simulink model "flightControlSystem"  (R2024a)
settings: Solver=ode3  StartTime=0  StopTime=TFinal  FixedStep=Ts  RelTol=1e-3  EnableMultiTasking=on
undefined symbols (not defined in the file): codertarget, Controller, DiscIntNeverNeededParam, Discrete, Estimator, g, init, orient_ref, pos_ref, Sensors, Time, Ts, var_acc_angle_N, var_bias_gyr_N, var_gyro_p_N, Vehicle
libraries: simulink x125, slpidlib x35, ctrlSharedLib x12, sharedtransform x10, eeGeneralControl x8, parrotlib x6, shareduavrstlib x1, simulink_need_slupdate x1
(part 9 of 11)

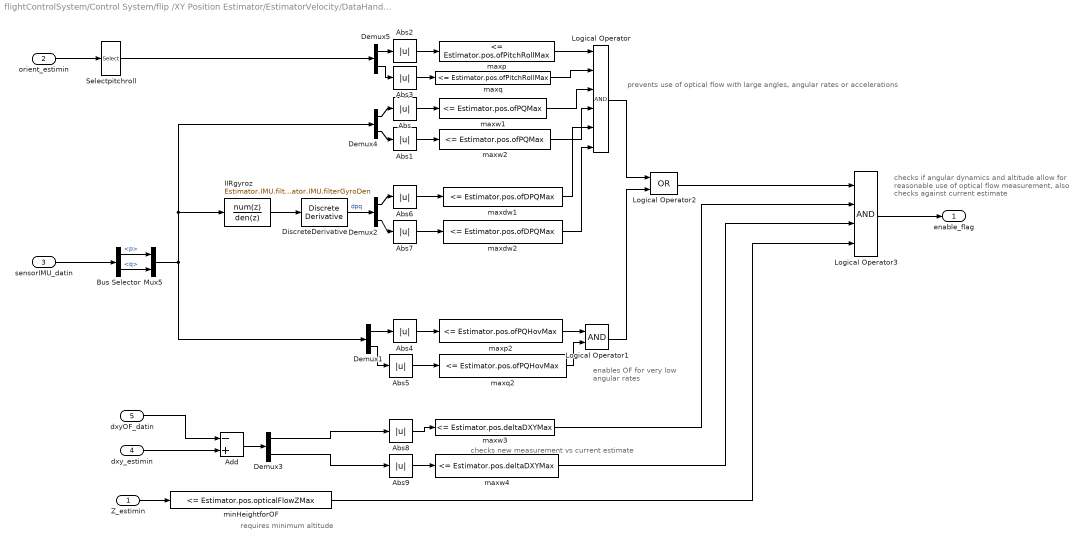
== system flightControlSystem/Control System/flip /XY Position Estimator/EstimatorVelocity/DataHandling ==
  note: prevents use of optical flow with large angles, angular rates or accelerations
  note: enables OF for very
      | low angular rates
  note: checks if angular dynamics and altitude allow for
      | reasonable use of optical flow measurement,
      | also checks against current estimate
  note: checks new measurement vs current estimate
  note: requires minimum altitude
  Z_estimin : Inport
  orient_estimin : Inport  Port=2
  sensorIMU_datin : Inport  Port=3
  dxy_estimin : Inport  Port=4
  dxyOF_datin : Inport  Port=5
  Abs{,1..9} (10 alike) : Abs  SaturateOnIntegerOverflow=off
  Add : Sum  Inputs=-+
  Bus Selector : BusSelector  OutputSignals=p,q
  Demux{1..5} (5 alike) : Demux  Outputs=2
  DiscreteDerivative : simulink/Discrete/Discrete Derivative  gainval=1.0  ICPrevScaledInput=0.0  OutMin=[]  OutMax=[]  OutDataType=fixdt(1, 16)  OutScaling=2^-10  DoSatur=off
  IIRgyroz : DiscreteFilter  Numerator=Estimator.IMU.filterGyroNum  Denominator=Estimator.IMU.filterGyroDen
  Logical Operator : Logic  Inputs=6  AllPortsSameDT=off  OutDataTypeStr=boolean
  Logical Operator1 : Logic  AllPortsSameDT=off  OutDataTypeStr=boolean
  Logical Operator2 : Logic  Operator=OR  AllPortsSameDT=off  OutDataTypeStr=boolean
  Logical Operator3 : Logic  Inputs=4  AllPortsSameDT=off  OutDataTypeStr=boolean
  Mux5 : Mux  Inputs=2
  Selectpitchroll : Selector  InputPortWidth=3  IndexOptions=Index vector (dialog)  Indices=[2 3]  OutputSizes=1
  maxdw1 : simulink/Logic and Bit Operations/Compare To Constant  relop=<=  const=Estimator.pos.ofDPQMax  OutDataTypeStr=boolean
  maxdw2 : simulink/Logic and Bit Operations/Compare To Constant  relop=<=  const=Estimator.pos.ofDPQMax  OutDataTypeStr=boolean
  maxp : simulink/Logic and Bit Operations/Compare To Constant  relop=<=  const=Estimator.pos.ofPitchRollMax  OutDataTypeStr=boolean
  maxp2 : simulink/Logic and Bit Operations/Compare To Constant  relop=<=  const=Estimator.pos.ofPQHovMax  OutDataTypeStr=boolean
  maxq : simulink/Logic and Bit Operations/Compare To Constant  relop=<=  const=Estimator.pos.ofPitchRollMax  OutDataTypeStr=boolean
  maxq2 : simulink/Logic and Bit Operations/Compare To Constant  relop=<=  const=Estimator.pos.ofPQHovMax  OutDataTypeStr=boolean
  maxw1 : simulink/Logic and Bit Operations/Compare To Constant  relop=<=  const=Estimator.pos.ofPQMax  OutDataTypeStr=boolean
  maxw2 : simulink/Logic and Bit Operations/Compare To Constant  relop=<=  const=Estimator.pos.ofPQMax  OutDataTypeStr=boolean
  maxw3 : simulink/Logic and Bit Operations/Compare To Constant  relop=<=  const=Estimator.pos.deltaDXYMax  OutDataTypeStr=boolean
  maxw4 : simulink/Logic and Bit Operations/Compare To Constant  relop=<=  const=Estimator.pos.deltaDXYMax  OutDataTypeStr=boolean
  minHeightforOF : simulink/Logic and Bit Operations/Compare To Constant  relop=<=  const=Estimator.pos.opticalFlowZMax  OutDataTypeStr=boolean
  enable_flag : Outport  VectorParamsAs1DForOutWhenUnconnected=off
  wires:
  minHeightforOF/1 -> Logical Operator3/4
  IIRgyroz/1 -> DiscreteDerivative/1
  Mux5/1 -> Demux1/1, Demux4/1, IIRgyroz/1
  maxw4/1 -> Logical Operator3/3
  maxw3/1 -> Logical Operator3/2
  dxyOF_datin/1 -> Add/1
  Demux3/2 -> Abs9/1
  Demux3/1 -> Abs8/1
  dxy_estimin/1 -> Add/2
  Add/1 -> Demux3/1
  Abs9/1 -> maxw4/1
  Abs8/1 -> maxw3/1
  Logical Operator2/1 -> Logical Operator3/1
  Logical Operator3/1 -> enable_flag/1
  DiscreteDerivative/1 -> Demux2/1  "dpq"
  Demux2/2 -> Abs7/1
  Demux2/1 -> Abs6/1
  Abs7/1 -> maxdw2/1
  Abs6/1 -> maxdw1/1
  Logical Operator1/1 -> Logical Operator2/2
  Demux1/2 -> Abs5/1
  Demux1/1 -> Abs4/1
  Abs5/1 -> maxq2/1
  Abs4/1 -> maxp2/1
  Abs3/1 -> maxq/1
  Abs2/1 -> maxp/1
  Demux4/2 -> Abs1/1
  Demux4/1 -> Abs/1
  Abs1/1 -> maxw2/1
  Abs/1 -> maxw1/1
  Z_estimin/1 -> minHeightforOF/1
  Logical Operator/1 -> Logical Operator2/1
  maxw1/1 -> Logical Operator/3
  Bus Selector/1 -> Mux5/1  "<p>"
  Selectpitchroll/1 -> Demux5/1
  sensorIMU_datin/1 -> Bus Selector/1
  maxq2/1 -> Logical Operator1/2
  Bus Selector/2 -> Mux5/2  "<q>"
  maxp/1 -> Logical Operator/1
  maxw2/1 -> Logical Operator/4
  orient_estimin/1 -> Selectpitchroll/1
  maxdw1/1 -> Logical Operator/5
  maxdw2/1 -> Logical Operator/6
  maxq/1 -> Logical Operator/2
  Demux5/1 -> Abs2/1
  Demux5/2 -> Abs3/1
  maxp2/1 -> Logical Operator1/1

== system flightControlSystem/Control System/flip /XY Position Estimator/EstimatorVelocity/XY velocity w//o angular velocity compensation ==
  note: Optical flow raw readings are converted to velocity in m/s based on the estimated altitude
  optical_flow : Inport
  z_estimate : Inport  Port=2
  " " : Product  Inputs=**
  Compare To Constant : simulink/Logic and Bit Operations/Compare To Constant  relop=<  const=200*4  OutDataTypeStr=boolean
  Counter Free-Running : simulink/Sources/Counter Free-Running  NumBits=32  tsamp=-1
  Gain : Gain  Gain=-1
  Select dxy : Selector  InputPortWidth=3  IndexOptions=Index vector (dialog)  Indices=[1 2]  OutputSizes=1
  Switch : Switch  Criteria=u2 > Threshold  SaturateOnIntegerOverflow=off  InputSameDT=off
  opticalFlowErrorCorrect : Gain  Gain=1.15
  optical_flow_dx_dy : Outport
  wires:
  Select dxy/1 -> optical_flow_dx_dy/1  "optical_flow_dx_dy"
  " "/1 -> opticalFlowErrorCorrect/1
  opticalFlowErrorCorrect/1 -> Switch/3
  Gain/1 -> " "/2
  Switch/1 -> Select dxy/1
  Counter Free-Running/1 -> Compare To Constant/1
  Compare To Constant/1 -> Switch/2
  optical_flow/1 -> " "/1, Switch/1
  z_estimate/1 -> Gain/1

== system flightControlSystem/Control System/normal/SensorPreprocessing/Temperature Compensation/Triggered Subsystem ==
  In1 : Inport
  Trigger : TriggerPort  TriggerType=either  VariantControl=Variant
  Out1 : Outport
  wires:
  In1/1 -> Out1/1

== system flightControlSystem/Control System/normal/XY Position Estimator/EstimatorVelocity/AccelerationHandling ==
  dxy_estimin : Inport
  sensorIMU_datin : Inport  Port=2
  orient_estimin : Inport  Port=3
  Z_estimin : Inport  Port=4
  Add : Sum  Inputs=-+
  Bus Selector1 : BusSelector  OutputSignals=ddx,ddy,ddz
  Deactivate Acceleration If OF is not used due to low altitude : simulink/Logic and Bit Operations/Compare To Constant  relop=<=  const=Estimator.pos.opticalFlowZMax  OutDataTypeStr=boolean
  Logical Operator : Logic  Operator=OR  AllPortsSameDT=off  OutDataTypeStr=boolean
  Mux6 : Mux  Inputs=3
  Product : Product  Inputs=3
  Product1 : Product  Multiplication=Matrix(*)
  Rotation Angles to Direction Cosine Matrix : sharedtransform/Rotation Angles to Direction Cosine Matrix  rotationOrder=ZYX  aMode=aMode
  SelectPlanarddxy : Selector  InputPortWidth=3  IndexOptions=Index vector (dialog)  Indices=[1 2]  OutputSizes=1
  Selector : Selector  InputPortWidth=2  IndexOptions=Index vector (dialog)  Indices=1  OutputSizes=1
  Selector1 : Selector  InputPortWidth=2  IndexOptions=Index vector (dialog)  Indices=2  OutputSizes=1
  do not use acc if optical flow never available (Note OF@60Hz but ZOH to 200!) : simulink/Logic and Bit Operations/Compare To Constant  relop=~=  const=0  OutDataTypeStr=boolean
  do not use acc if optical flow never available (Note OF@60Hz but ZOH to 200!)1 : simulink/Logic and Bit Operations/Compare To Constant  relop=~=  const=0  OutDataTypeStr=boolean
  gainaccinput1 : Gain  OutDataTypeStr=single
  gravity : Constant  Value=[0 0 -g]
  acceleration_world : Outport  OutDataTypeStr=single  VectorParamsAs1DForOutWhenUnconnected=off
  wires:
  do not use acc if optical flow never available (Note OF@60Hz but ZOH to 200!)1/1 -> Logical Operator/2
  do not use acc if optical flow never available (Note OF@60Hz but ZOH to 200!)/1 -> Logical Operator/1
  Logical Operator/1 -> Product/1
  Selector1/1 -> do not use acc if optical flow never available (Note OF@60Hz but ZOH to 200!)1/1
  Selector/1 -> do not use acc if optical flow never available (Note OF@60Hz but ZOH to 200!)/1
  dxy_estimin/1 -> Selector1/1, Selector/1
  Product/1 -> acceleration_world/1
  Deactivate Acceleration If OF is not used due to low altitude/1 -> Product/3
  Z_estimin/1 -> Deactivate Acceleration If OF is not used due to low altitude/1
  Add/1 -> SelectPlanarddxy/1
  Product1/1 -> Add/1
  gravity/1 -> Product1/2
  SelectPlanarddxy/1 -> gainaccinput1/1
  Bus Selector1/3 -> Mux6/3  "<ddz>"
  Bus Selector1/1 -> Mux6/1  "<ddx>"
  sensorIMU_datin/1 -> Bus Selector1/1
  Mux6/1 -> Add/2
  Bus Selector1/2 -> Mux6/2  "<ddy>"
  orient_estimin/1 -> Rotation Angles to Direction Cosine Matrix/1
  Rotation Angles to Direction Cosine Matrix/1 -> Product1/1
  gainaccinput1/1 -> Product/2

== system flightControlSystem/Control System/normal/XY Position Estimator/EstimatorVelocity/Angular velocity compensation for optical flow ==
  note: Optical flow readings are affected by both linear and angular velocity of the drone. We need to subtract the effect of angular velocity before using the flow data
  z_estimate : Inport
  Angular velocity w/o bias : Inport  Port=2
  Abs : Abs  SaturateOnIntegerOverflow=off
  Data Type Conversion : DataTypeConversion  SaturateOnIntegerOverflow=off  RndMeth=Floor
  Demux : Demux  Outputs=2
  Gain1 : Gain  Gain=-1
  Mux : Mux  Inputs=2
  Selector : Selector  InputPortWidth=3  IndexOptions=Index vector (dialog)  Indices=[1 2]  OutputSizes=1
  prod : Product  Inputs=**
  angular velocity correction : Outport
  wires:
  Gain1/1 -> Mux/1
  Mux/1 -> Data Type Conversion/1
  Demux/2 -> Gain1/1
  Data Type Conversion/1 -> angular velocity correction/1
  prod/1 -> Demux/1
  z_estimate/1 -> Abs/1
  Demux/1 -> Mux/2
  Selector/1 -> prod/2
  Abs/1 -> prod/1
  Angular velocity w/o bias/1 -> Selector/1

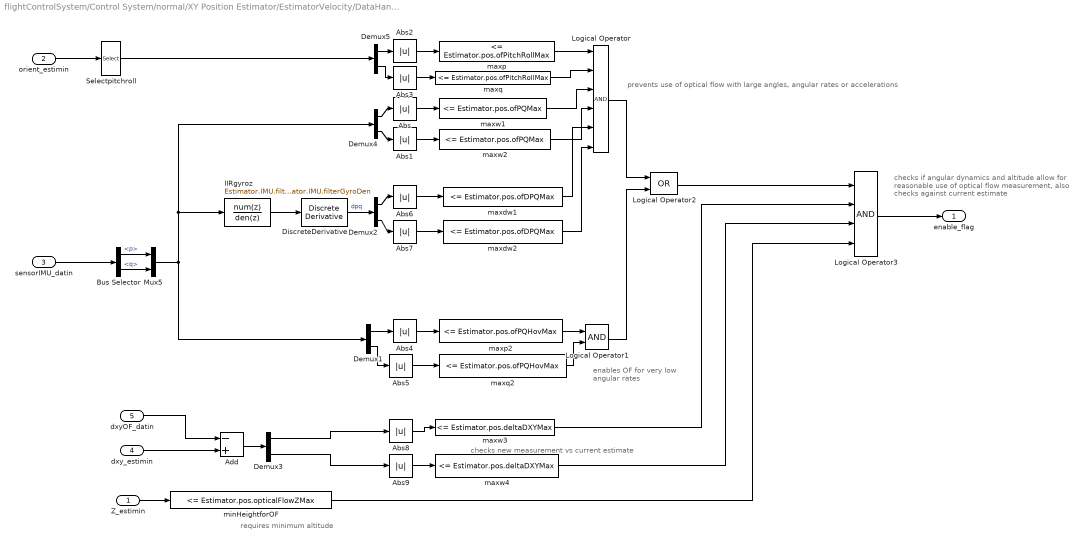
== system flightControlSystem/Control System/normal/XY Position Estimator/EstimatorVelocity/DataHandling ==
  note: prevents use of optical flow with large angles, angular rates or accelerations
  note: enables OF for very
      | low angular rates
  note: checks if angular dynamics and altitude allow for
      | reasonable use of optical flow measurement,
      | also checks against current estimate
  note: checks new measurement vs current estimate
  note: requires minimum altitude
  Z_estimin : Inport
  orient_estimin : Inport  Port=2
  sensorIMU_datin : Inport  Port=3
  dxy_estimin : Inport  Port=4
  dxyOF_datin : Inport  Port=5
  Abs{,1..9} (10 alike) : Abs  SaturateOnIntegerOverflow=off
  Add : Sum  Inputs=-+
  Bus Selector : BusSelector  OutputSignals=p,q
  Demux{1..5} (5 alike) : Demux  Outputs=2
  DiscreteDerivative : simulink/Discrete/Discrete Derivative  gainval=1.0  ICPrevScaledInput=0.0  OutMin=[]  OutMax=[]  OutDataType=fixdt(1, 16)  OutScaling=2^-10  DoSatur=off
  IIRgyroz : DiscreteFilter  Numerator=Estimator.IMU.filterGyroNum  Denominator=Estimator.IMU.filterGyroDen
  Logical Operator : Logic  Inputs=6  AllPortsSameDT=off  OutDataTypeStr=boolean
  Logical Operator1 : Logic  AllPortsSameDT=off  OutDataTypeStr=boolean
  Logical Operator2 : Logic  Operator=OR  AllPortsSameDT=off  OutDataTypeStr=boolean
  Logical Operator3 : Logic  Inputs=4  AllPortsSameDT=off  OutDataTypeStr=boolean
  Mux5 : Mux  Inputs=2
  Selectpitchroll : Selector  InputPortWidth=3  IndexOptions=Index vector (dialog)  Indices=[2 3]  OutputSizes=1
  maxdw1 : simulink/Logic and Bit Operations/Compare To Constant  relop=<=  const=Estimator.pos.ofDPQMax  OutDataTypeStr=boolean
  maxdw2 : simulink/Logic and Bit Operations/Compare To Constant  relop=<=  const=Estimator.pos.ofDPQMax  OutDataTypeStr=boolean
  maxp : simulink/Logic and Bit Operations/Compare To Constant  relop=<=  const=Estimator.pos.ofPitchRollMax  OutDataTypeStr=boolean
  maxp2 : simulink/Logic and Bit Operations/Compare To Constant  relop=<=  const=Estimator.pos.ofPQHovMax  OutDataTypeStr=boolean
  maxq : simulink/Logic and Bit Operations/Compare To Constant  relop=<=  const=Estimator.pos.ofPitchRollMax  OutDataTypeStr=boolean
  maxq2 : simulink/Logic and Bit Operations/Compare To Constant  relop=<=  const=Estimator.pos.ofPQHovMax  OutDataTypeStr=boolean
  maxw1 : simulink/Logic and Bit Operations/Compare To Constant  relop=<=  const=Estimator.pos.ofPQMax  OutDataTypeStr=boolean
  maxw2 : simulink/Logic and Bit Operations/Compare To Constant  relop=<=  const=Estimator.pos.ofPQMax  OutDataTypeStr=boolean
  maxw3 : simulink/Logic and Bit Operations/Compare To Constant  relop=<=  const=Estimator.pos.deltaDXYMax  OutDataTypeStr=boolean
  maxw4 : simulink/Logic and Bit Operations/Compare To Constant  relop=<=  const=Estimator.pos.deltaDXYMax  OutDataTypeStr=boolean
  minHeightforOF : simulink/Logic and Bit Operations/Compare To Constant  relop=<=  const=Estimator.pos.opticalFlowZMax  OutDataTypeStr=boolean
  enable_flag : Outport  VectorParamsAs1DForOutWhenUnconnected=off
  wires:
  minHeightforOF/1 -> Logical Operator3/4
  IIRgyroz/1 -> DiscreteDerivative/1
  Mux5/1 -> Demux1/1, Demux4/1, IIRgyroz/1
  maxw4/1 -> Logical Operator3/3
  maxw3/1 -> Logical Operator3/2
  dxyOF_datin/1 -> Add/1
  Demux3/2 -> Abs9/1
  Demux3/1 -> Abs8/1
  dxy_estimin/1 -> Add/2
  Add/1 -> Demux3/1
  Abs9/1 -> maxw4/1
  Abs8/1 -> maxw3/1
  Logical Operator2/1 -> Logical Operator3/1
  Logical Operator3/1 -> enable_flag/1
  DiscreteDerivative/1 -> Demux2/1  "dpq"
  Demux2/2 -> Abs7/1
  Demux2/1 -> Abs6/1
  Abs7/1 -> maxdw2/1
  Abs6/1 -> maxdw1/1
  Logical Operator1/1 -> Logical Operator2/2
  Demux1/2 -> Abs5/1
  Demux1/1 -> Abs4/1
  Abs5/1 -> maxq2/1
  Abs4/1 -> maxp2/1
  Abs3/1 -> maxq/1
  Abs2/1 -> maxp/1
  Demux4/2 -> Abs1/1
  Demux4/1 -> Abs/1
  Abs1/1 -> maxw2/1
  Abs/1 -> maxw1/1
  Z_estimin/1 -> minHeightforOF/1
  Logical Operator/1 -> Logical Operator2/1
  maxw1/1 -> Logical Operator/3
  Bus Selector/1 -> Mux5/1  "<p>"
  Selectpitchroll/1 -> Demux5/1
  sensorIMU_datin/1 -> Bus Selector/1
  maxq2/1 -> Logical Operator1/2
  Bus Selector/2 -> Mux5/2  "<q>"
  maxp/1 -> Logical Operator/1
  maxw2/1 -> Logical Operator/4
  orient_estimin/1 -> Selectpitchroll/1
  maxdw1/1 -> Logical Operator/5
  maxdw2/1 -> Logical Operator/6
  maxq/1 -> Logical Operator/2
  Demux5/1 -> Abs2/1
  Demux5/2 -> Abs3/1
  maxp2/1 -> Logical Operator1/1

== system flightControlSystem/Control System/normal/XY Position Estimator/EstimatorVelocity/xy velocity w//o angular velocity compensation ==
  note: Optical flow raw readings are converted to velocity in m/s based on the estimated altitude
  optical_flow : Inport
  z_estimate : Inport  Port=2
  " " : Product  Inputs=**
  Compare To Constant : simulink/Logic and Bit Operations/Compare To Constant  relop=<  const=200*4  OutDataTypeStr=boolean
  Counter Free-Running : simulink/Sources/Counter Free-Running  NumBits=32  tsamp=-1
  Gain : Gain  Gain=-1
  Select dxy : Selector  InputPortWidth=3  IndexOptions=Index vector (dialog)  Indices=[1 2]  OutputSizes=1
  Switch : Switch  Criteria=u2 > Threshold  SaturateOnIntegerOverflow=off  InputSameDT=off
  opticalFlowErrorCorrect : Gain  Gain=1.15
  optical_flow_dx_dy : Outport
  wires:
  Select dxy/1 -> optical_flow_dx_dy/1  "optical_flow_dx_dy"
  " "/1 -> opticalFlowErrorCorrect/1
  opticalFlowErrorCorrect/1 -> Switch/3
  Gain/1 -> " "/2
  Switch/1 -> Select dxy/1
  Counter Free-Running/1 -> Compare To Constant/1
  Compare To Constant/1 -> Switch/2
  optical_flow/1 -> " "/1, Switch/1
  z_estimate/1 -> Gain/1

== system flightControlSystem/Flight Control System/State Estimator/SensorPreprocessing/Temperature Compensation/Triggered Subsystem ==
  In1 : Inport
  Trigger : TriggerPort  TriggerType=either  VariantControl=Variant
  Out1 : Outport
  wires:
  In1/1 -> Out1/1

== system flightControlSystem/Flight Control System/State Estimator/XY Position Estimator/EstimatorVelocity/AccelerationHandling ==
  dxy_estimin : Inport
  sensorIMU_datin : Inport  Port=2
  orient_estimin : Inport  Port=3
  Z_estimin : Inport  Port=4
  Add : Sum  Inputs=-+
  Bus Selector1 : BusSelector  OutputSignals=ddx,ddy,ddz
  Deactivate Acceleration If OF is not used due to low altitude : simulink/Logic and Bit Operations/Compare To Constant  relop=<=  const=Estimator.pos.opticalFlowZMax  OutDataTypeStr=boolean
  Logical Operator : Logic  Operator=OR  AllPortsSameDT=off  OutDataTypeStr=boolean
  Mux6 : Mux  Inputs=3
  Product : Product  Inputs=3
  Product1 : Product  Multiplication=Matrix(*)
  Rotation Angles to Direction Cosine Matrix : sharedtransform/Rotation Angles to Direction Cosine Matrix  rotationOrder=ZYX  aMode=aMode
  SelectPlanarddxy : Selector  InputPortWidth=3  IndexOptions=Index vector (dialog)  Indices=[1 2]  OutputSizes=1
  Selector : Selector  InputPortWidth=2  IndexOptions=Index vector (dialog)  Indices=1  OutputSizes=1
  Selector1 : Selector  InputPortWidth=2  IndexOptions=Index vector (dialog)  Indices=2  OutputSizes=1
  do not use acc if optical flow never available (Note OF@60Hz but ZOH to 200!) : simulink/Logic and Bit Operations/Compare To Constant  relop=~=  const=0  OutDataTypeStr=boolean
  do not use acc if optical flow never available (Note OF@60Hz but ZOH to 200!)1 : simulink/Logic and Bit Operations/Compare To Constant  relop=~=  const=0  OutDataTypeStr=boolean
  gainaccinput1 : Gain  OutDataTypeStr=single
  gravity : Constant  Value=[0 0 -g]
  acceleration_world : Outport  OutDataTypeStr=single  VectorParamsAs1DForOutWhenUnconnected=off
  wires:
  do not use acc if optical flow never available (Note OF@60Hz but ZOH to 200!)1/1 -> Logical Operator/2
  do not use acc if optical flow never available (Note OF@60Hz but ZOH to 200!)/1 -> Logical Operator/1
  Logical Operator/1 -> Product/1
  Selector1/1 -> do not use acc if optical flow never available (Note OF@60Hz but ZOH to 200!)1/1
  Selector/1 -> do not use acc if optical flow never available (Note OF@60Hz but ZOH to 200!)/1
  dxy_estimin/1 -> Selector1/1, Selector/1
  Product/1 -> acceleration_world/1
  Deactivate Acceleration If OF is not used due to low altitude/1 -> Product/3
  Z_estimin/1 -> Deactivate Acceleration If OF is not used due to low altitude/1
  Add/1 -> SelectPlanarddxy/1
  Product1/1 -> Add/1
  gravity/1 -> Product1/2
  SelectPlanarddxy/1 -> gainaccinput1/1
  Bus Selector1/3 -> Mux6/3  "<ddz>"
  Bus Selector1/1 -> Mux6/1  "<ddx>"
  sensorIMU_datin/1 -> Bus Selector1/1
  Mux6/1 -> Add/2
  Bus Selector1/2 -> Mux6/2  "<ddy>"
  orient_estimin/1 -> Rotation Angles to Direction Cosine Matrix/1
  Rotation Angles to Direction Cosine Matrix/1 -> Product1/1
  gainaccinput1/1 -> Product/2

== system flightControlSystem/Flight Control System/State Estimator/XY Position Estimator/EstimatorVelocity/Angular velocity compensation for optical flow ==
  note: Optical flow readings are affected by both linear and angular velocity of the drone. We need to subtract the effect of angular velocity before using the flow data
  z_estimate : Inport
  Angular velocity w/o bias : Inport  Port=2
  Abs : Abs  SaturateOnIntegerOverflow=off
  Data Type Conversion : DataTypeConversion  SaturateOnIntegerOverflow=off  RndMeth=Floor
  Demux : Demux  Outputs=2
  Gain1 : Gain  Gain=-1
  Mux : Mux  Inputs=2
  Selector : Selector  InputPortWidth=3  IndexOptions=Index vector (dialog)  Indices=[1 2]  OutputSizes=1
  prod : Product  Inputs=**
  angular velocity correction : Outport
  wires:
  Gain1/1 -> Mux/1
  Mux/1 -> Data Type Conversion/1
  Demux/2 -> Gain1/1
  Data Type Conversion/1 -> angular velocity correction/1
  prod/1 -> Demux/1
  z_estimate/1 -> Abs/1
  Demux/1 -> Mux/2
  Selector/1 -> prod/2
  Abs/1 -> prod/1
  Angular velocity w/o bias/1 -> Selector/1

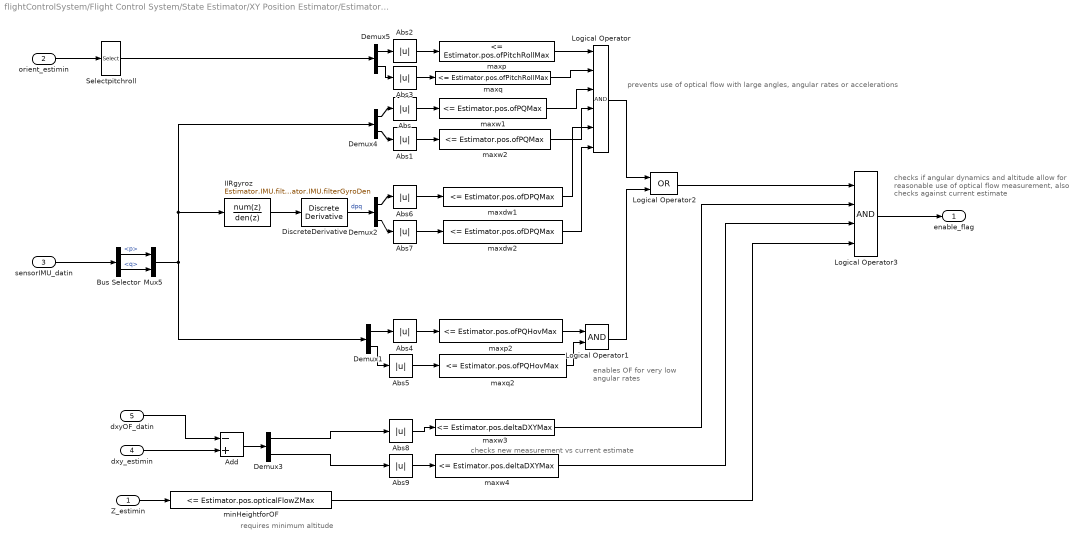
== system flightControlSystem/Flight Control System/State Estimator/XY Position Estimator/EstimatorVelocity/DataHandling ==
  note: prevents use of optical flow with large angles, angular rates or accelerations
  note: enables OF for very
      | low angular rates
  note: checks if angular dynamics and altitude allow for
      | reasonable use of optical flow measurement,
      | also checks against current estimate
  note: checks new measurement vs current estimate
  note: requires minimum altitude
  Z_estimin : Inport
  orient_estimin : Inport  Port=2
  sensorIMU_datin : Inport  Port=3
  dxy_estimin : Inport  Port=4
  dxyOF_datin : Inport  Port=5
  Abs{,1..9} (10 alike) : Abs  SaturateOnIntegerOverflow=off
  Add : Sum  Inputs=-+
  Bus Selector : BusSelector  OutputSignals=p,q
  Demux{1..5} (5 alike) : Demux  Outputs=2
  DiscreteDerivative : simulink/Discrete/Discrete Derivative  gainval=1.0  ICPrevScaledInput=0.0  OutMin=[]  OutMax=[]  OutDataType=fixdt(1, 16)  OutScaling=2^-10  DoSatur=off
  IIRgyroz : DiscreteFilter  Numerator=Estimator.IMU.filterGyroNum  Denominator=Estimator.IMU.filterGyroDen
  Logical Operator : Logic  Inputs=6  AllPortsSameDT=off  OutDataTypeStr=boolean
  Logical Operator1 : Logic  AllPortsSameDT=off  OutDataTypeStr=boolean
  Logical Operator2 : Logic  Operator=OR  AllPortsSameDT=off  OutDataTypeStr=boolean
  Logical Operator3 : Logic  Inputs=4  AllPortsSameDT=off  OutDataTypeStr=boolean
  Mux5 : Mux  Inputs=2
  Selectpitchroll : Selector  InputPortWidth=3  IndexOptions=Index vector (dialog)  Indices=[2 3]  OutputSizes=1
  maxdw1 : simulink/Logic and Bit Operations/Compare To Constant  relop=<=  const=Estimator.pos.ofDPQMax  OutDataTypeStr=boolean
  maxdw2 : simulink/Logic and Bit Operations/Compare To Constant  relop=<=  const=Estimator.pos.ofDPQMax  OutDataTypeStr=boolean
  maxp : simulink/Logic and Bit Operations/Compare To Constant  relop=<=  const=Estimator.pos.ofPitchRollMax  OutDataTypeStr=boolean
  maxp2 : simulink/Logic and Bit Operations/Compare To Constant  relop=<=  const=Estimator.pos.ofPQHovMax  OutDataTypeStr=boolean
  maxq : simulink/Logic and Bit Operations/Compare To Constant  relop=<=  const=Estimator.pos.ofPitchRollMax  OutDataTypeStr=boolean
  maxq2 : simulink/Logic and Bit Operations/Compare To Constant  relop=<=  const=Estimator.pos.ofPQHovMax  OutDataTypeStr=boolean
  maxw1 : simulink/Logic and Bit Operations/Compare To Constant  relop=<=  const=Estimator.pos.ofPQMax  OutDataTypeStr=boolean
  maxw2 : simulink/Logic and Bit Operations/Compare To Constant  relop=<=  const=Estimator.pos.ofPQMax  OutDataTypeStr=boolean
  maxw3 : simulink/Logic and Bit Operations/Compare To Constant  relop=<=  const=Estimator.pos.deltaDXYMax  OutDataTypeStr=boolean
  maxw4 : simulink/Logic and Bit Operations/Compare To Constant  relop=<=  const=Estimator.pos.deltaDXYMax  OutDataTypeStr=boolean
  minHeightforOF : simulink/Logic and Bit Operations/Compare To Constant  relop=<=  const=Estimator.pos.opticalFlowZMax  OutDataTypeStr=boolean
  enable_flag : Outport  VectorParamsAs1DForOutWhenUnconnected=off
  wires:
  minHeightforOF/1 -> Logical Operator3/4
  IIRgyroz/1 -> DiscreteDerivative/1
  Mux5/1 -> Demux1/1, Demux4/1, IIRgyroz/1
  maxw4/1 -> Logical Operator3/3
  maxw3/1 -> Logical Operator3/2
  dxyOF_datin/1 -> Add/1
  Demux3/2 -> Abs9/1
  Demux3/1 -> Abs8/1
  dxy_estimin/1 -> Add/2
  Add/1 -> Demux3/1
  Abs9/1 -> maxw4/1
  Abs8/1 -> maxw3/1
  Logical Operator2/1 -> Logical Operator3/1
  Logical Operator3/1 -> enable_flag/1
  DiscreteDerivative/1 -> Demux2/1  "dpq"
  Demux2/2 -> Abs7/1
  Demux2/1 -> Abs6/1
  Abs7/1 -> maxdw2/1
  Abs6/1 -> maxdw1/1
  Logical Operator1/1 -> Logical Operator2/2
  Demux1/2 -> Abs5/1
  Demux1/1 -> Abs4/1
  Abs5/1 -> maxq2/1
  Abs4/1 -> maxp2/1
  Abs3/1 -> maxq/1
  Abs2/1 -> maxp/1
  Demux4/2 -> Abs1/1
  Demux4/1 -> Abs/1
  Abs1/1 -> maxw2/1
  Abs/1 -> maxw1/1
  Z_estimin/1 -> minHeightforOF/1
  Logical Operator/1 -> Logical Operator2/1
  maxw1/1 -> Logical Operator/3
  Bus Selector/1 -> Mux5/1  "<p>"
  Selectpitchroll/1 -> Demux5/1
  sensorIMU_datin/1 -> Bus Selector/1
  maxq2/1 -> Logical Operator1/2
  Bus Selector/2 -> Mux5/2  "<q>"
  maxp/1 -> Logical Operator/1
  maxw2/1 -> Logical Operator/4
  orient_estimin/1 -> Selectpitchroll/1
  maxdw1/1 -> Logical Operator/5
  maxdw2/1 -> Logical Operator/6
  maxq/1 -> Logical Operator/2
  Demux5/1 -> Abs2/1
  Demux5/2 -> Abs3/1
  maxp2/1 -> Logical Operator1/1

== system flightControlSystem/Flight Control System/State Estimator/XY Position Estimator/EstimatorVelocity/xy velocity w//o angular velocity compensation ==
  note: Optical flow raw readings are converted to velocity in m/s based on the estimated altitude
  optical_flow : Inport
  z_estimate : Inport  Port=2
  " " : Product  Inputs=**
  Compare To Constant : simulink/Logic and Bit Operations/Compare To Constant  relop=<  const=200*4  OutDataTypeStr=boolean
  Counter Free-Running : simulink/Sources/Counter Free-Running  NumBits=32  tsamp=-1
  Gain : Gain  Gain=-1
  Select dxy : Selector  InputPortWidth=3  IndexOptions=Index vector (dialog)  Indices=[1 2]  OutputSizes=1
  Switch : Switch  Criteria=u2 > Threshold  SaturateOnIntegerOverflow=off  InputSameDT=off
  opticalFlowErrorCorrect : Gain  Gain=1.15
  optical_flow_dx_dy : Outport
  wires:
  Select dxy/1 -> optical_flow_dx_dy/1  "optical_flow_dx_dy"
  " "/1 -> opticalFlowErrorCorrect/1
  opticalFlowErrorCorrect/1 -> Switch/3
  Gain/1 -> " "/2
  Switch/1 -> Select dxy/1
  Counter Free-Running/1 -> Compare To Constant/1
  Compare To Constant/1 -> Switch/2
  optical_flow/1 -> " "/1, Switch/1
  z_estimate/1 -> Gain/1

== matlab function flightControlSystem/Control System/flip /Attitude Estimator/MATLAB Function1 ==
  data: acc input; q output; gyro input; prevQuat input
function q = fcn(acc, gyro, prevQuat)
    
    
    kcorr = 0.002;
    
    w = norm(gyro);
    
    sigmaW = 0.5 * [0 -gyro';...
        gyro(1) 0 gyro(3) -gyro(2);...
        gyro(2) -gyro(3) 0 gyro(1);...
        gyro(3) gyro(2) -gyro(1) 0];
    
    if w==0
        qpred = prevQuat;
    else
        qpred = (eye(4)*cos(w*0.0025) + (2/w)* sigmaW * sin(w*0.0025))*prevQuat;
    end
    
    if (w < 1) && (abs(norm(acc)-9.81) < 2.9)
        
        qpred = quaternion(qpred');

        accW = rotateframe(conj(qpred),acc');
        
        accW = accW/norm(accW);
        
        epred = [0,0,-1];

        beta = acos(epred*accW');

        hB = cross(accW',epred');

        hB = hB / norm(hB);

        qcorr = quaternion([cos(kcorr*beta/2), hB'*sin(kcorr*beta/2)]);

        qpred = qcorr * qpred;

        [a,b,c,d] = qpred.parts;
        
        qpred = [a,b,c,d]';
    end
    
q =  qpred;
end

== matlab function flightControlSystem/Control System/flip/MATLAB Function ==
  data: t input; w_d output; ap_ input
function w_d = fcn(t, ap_)

w_d = 0;
wmax = 1600*pi/180;
% g1 = pi/wmax;
% b1 = -3/4 * wmax;
% 
% if t > 10 && t < 10.25
%     w_d = (t-10) * wmax/0.25;
% elseif t >= 10.25 && t < 10.5
%     w_d = -(t-10)*wmax/0.25 + 2*wmax;
% end


if t > 10 && t < 10.2287
    w_d = wmax;
elseif t >= 10.2287 && t < 10.2856
    w_d = -(t-10)*wmax/0.0569 + 5.0193*wmax;
end

if ap_ > 360
    w_d = 0;
end

== matlab function flightControlSystem/Control System/flip/Position Controller/Position error transformation (Earth to Body frame) ==
  data: yaw input; xy_err_earth input; xy_err_body output
function xy_err_body = fcn(yaw,xy_err_earth)

transformation = [cos(yaw), sin(yaw); -sin(yaw),  cos(yaw)];
xy_err_body = transformation * xy_err_earth;


end

== matlab function flightControlSystem/Control System/Path Planning/Subsystem3/MATLAB Function2 ==
  data: data input; x_new input; xdd_des output; y_new input; xd_new input; yd_new input; ydd_des output; xdd_new input; ydd_new input; x input; y input; dx input; dy input; ddx input; ddy input
function [xdd_des, ydd_des] = fcn(data, x_new, y_new, xd_new, yd_new, xdd_new, ydd_new, x, y, dx, dy, ddx, ddy)
    % PID gains
    kpx = single(0.0001);
    kpy = single(0.0001);
    kdx = single(0.00001);
    kdy = single(0.00001);

    % Compute desired accelerations
    xdd_des = single(0.0000031 * (xdd_new - ddx) + kdx * (xd_new - dx) + kpx * (x_new - x));
    ydd_des = single(0.0000031 * (ydd_new - ddy) + kdy * (yd_new - dy) + kpy * (y_new - y));
end

== matlab function flightControlSystem/Control System/Path Planning/Subsystem3/MATLAB Function3 ==
  data: xdd_des input; phi_des output; ydd_des input; psi input; theta_des output
function [phi_des, theta_des] = fcn(xdd_des, ydd_des, psi)
    g = 9.81;
    phi_des = single(1/g * (xdd_des * sin(psi) - ydd_des * cos(psi)));
    theta_des = single(-1/g * (xdd_des * cos(psi) + ydd_des * sin(psi)));
end

== stateflow chart flightControlSystem/Control System/Path Planning/Subsystem3/Chart1 ==
  state Hover
    entry:
    phi=0.0;
    theta=0.0;
  state phi_des
    phi=phi_des
    theta=theta_des
  (default) -> Hover
  Hover -> phi_des : [after(2,sec)]
  data: theta_des input; phi_des input; phi output double; theta output double

== stateflow chart flightControlSystem/Control System/Path Planning/Chart1 ==
  state MoveStraight
    during:
    xout=xout+0.006*x_new
    yout=yout+0.006*y_new
    zout=zout;
  state Hover
    entry:
    xout=0.0;
    yout=0.0;
    zout=-0.8;
  state MoveStraight4
    during:
    xout=xout+0.006*x_new;
    yout=yout+0.006*y_new;
    zout=zout+0.0000014*(sum_pixels)
  state land
    finaland=1
  (default) -> Hover
  Hover -> MoveStraight : [after(2,sec)]
  MoveStraight -> MoveStraight4 : [sum_pixels>60&&centroid_dist<25]
  MoveStraight4 -> land : [ zout>-0.4]
  data: ang input; sum_pixels input; centroid_dist input; forward input; right input; left input; sum_pix2 input; xestim input; yestim input; y_new input; xout output single; yout output single; zout output single; x_new input; dy input; dx input; s local; finaland output

== matlab function flightControlSystem/Control System/Path Planning/MATLAB Function2 ==
  data: u input; forward output; right output
function [forward,right]= fcn(u)

forward = u(1);
right=u(2);

== matlab function flightControlSystem/Control System/Controller/Position Controller/MATLAB Function1 ==
  data: ddx input; ddy input; ddx_filtered output; ddz input; ddy_filtered output; ddz_filtered output
function [ddx_filtered, ddy_filtered, ddz_filtered] = fcn(ddx, ddy, ddz)
    persistent filterInitialized b a;
    noise_margin = 0.005; % Define the margin around zero to be considered as noise
    
    if isempty(filterInitialized)
        % Design the filter according to your specifications
        % Example: 2nd-order Butterworth low-pass filter with a cutoff frequency of 5 Hz and a sample rate of 100 Hz
        
        [b, a] = butter(2, (7/(100/2)), 'low');
        filterInitialized = true;
    end
    
    % Apply the filter to each acceleration component
    ddx_temp = filter(b, a, ddx);
    ddy_temp = filter(b, a, ddy);
    ddz_temp = filter(b, a, ddz);

    % Apply the bias correction (deadzone)
    ddx_filtered = applyDeadzone(ddx_temp, noise_margin);
    ddy_filtered = applyDeadzone(ddy_temp, noise_margin);
    ddz_filtered = applyDeadzone(ddz_temp, noise_margin);
end

function val_filtered = applyDeadzone(val, margin)
    % Ensure that the function outputs the same type as the input
    if abs(val) < margin
        val_filtered = cast(0, 'like', val); % Cast zero to the type of val
    else
        val_filtered = val;
    end
end

== matlab function flightControlSystem/Control System/Controller/Position Controller/Position error transformation (Earth to Body frame)1 ==
  data: yaw input; xy_err_earth input; xy_err_body output
function xy_err_body = fcn(yaw,xy_err_earth)

transformation = [cos(yaw), sin(yaw); -sin(yaw),  cos(yaw)];
xy_err_body = transformation * xy_err_earth;


end

== matlab function flightControlSystem/Control System/Controller/Position Controller/Subsystem/MATLAB Function2 ==
  data: Xe input; xdd_des output; Ve input; Ae input; qd input; ydd_des output; q input; qdd input; Je input; qddd input
function [xdd_des, ydd_des] = fcn(Xe,Ve,Ae,qd,q,qdd, Je, qddd)


%Xe actual position x y z
%Ve ACtual velocity Ve(1) Ve(2) Ve(3)
%k2;dx=  kpz=

kpx=1.77;
kpy=1.77;
kpz=75;

kdx=3.4
kdy=3.4
kdz=45

kax=0.01;
kay=0.01;
kaz=0.01;

kjx=0.0002;
kjy=0.0002;
kjz=0.0002;

xdd_des=kjx*(qddd(1))+kax*(qdd(1)-Ae(1))+kdx*(qd(1)-Ve(1))+kpx*(q(1)-Xe(1))
ydd_des=kjy*(qddd(2))+kay*(qdd(2)-Ae(2))+kdy*(qd(2)-Ve(2))+kpy*(q(2)-Xe(2))
%zdd_des=kjz*(qddd(3))+kaz*(qdd(3)-Ae(3))+kdz*(qd(3)-Ve(3))+kpz*(q(3)-Xe(3))



end

== matlab function flightControlSystem/Control System/Controller/Position Controller/Subsystem/MATLAB Function3 ==
  data: u input; y output; u1 input; time input; t output
function [y ,t]= fcn(u, u1, time)



y=[u(1) u1(1);u(2) u1(2) ; u(3) u1(3)]

t=[time time+0.05]
 
end

== matlab function flightControlSystem/Control System/Controller/Position Controller/MATLAB Function2 ==
  data: ddx input; ddy input; ddx_filtered output; ddz input; ddy_filtered output; ddz_filtered output
function [ddx_filtered, ddy_filtered, ddz_filtered] = fcn(ddx, ddy, ddz)
    persistent filterInitialized b a;
    noise_margin = 0.005; % Define the margin around zero to be considered as noise
    
    if isempty(filterInitialized)
        % Design the filter according to your specifications
        % Example: 2nd-order Butterworth low-pass filter with a cutoff frequency of 5 Hz and a sample rate of 100 Hz
        
        [b, a] = butter(2, (7/(100/2)), 'low');
        filterInitialized = true;
    end
    
    % Apply the filter to each acceleration component
    ddx_temp = filter(b, a, ddx);
    ddy_temp = filter(b, a, ddy);
    ddz_temp = filter(b, a, ddz);

    % Apply the bias correction (deadzone)
    ddx_filtered = applyDeadzone(ddx_temp, noise_margin);
    ddy_filtered = applyDeadzone(ddy_temp, noise_margin);
    ddz_filtered = applyDeadzone(ddz_temp, noise_margin);
end

function val_filtered = applyDeadzone(val, margin)
    % Ensure that the function outputs the same type as the input
    if abs(val) < margin
        val_filtered = cast(0, 'like', val); % Cast zero to the type of val
    else
        val_filtered = val;
    end
end

== matlab function flightControlSystem/Control System/Controller/Position Controller/Position error transformation (Earth to Body frame)2 ==
  data: yaw input; xy_err_earth input; xy_err_body output
function xy_err_body = fcn(yaw,xy_err_earth)

transformation = [cos(yaw), sin(yaw); -sin(yaw),  cos(yaw)];
xy_err_body = transformation * xy_err_earth;


end

== matlab function flightControlSystem/Control System/Controller/Position Controller/MATLAB Function3 ==
  data: ddx input; ddy input; ddx_filtered output; ddz input; ddy_filtered output; ddz_filtered output
function [ddx_filtered, ddy_filtered, ddz_filtered] = fcn(ddx, ddy, ddz)
    persistent filterInitialized b a;
    noise_margin = 0.005; % Define the margin around zero to be considered as noise
    
    if isempty(filterInitialized)
        % Design the filter according to your specifications
        % Example: 2nd-order Butterworth low-pass filter with a cutoff frequency of 5 Hz and a sample rate of 100 Hz
        
        [b, a] = butter(2, (7/(100/2)), 'low');
        filterInitialized = true;
    end
    
    % Apply the filter to each acceleration component
    ddx_temp = filter(b, a, ddx);
    ddy_temp = filter(b, a, ddy);
    ddz_temp = filter(b, a, ddz);

    % Apply the bias correction (deadzone)
    ddx_filtered = applyDeadzone(ddx_temp, noise_margin);
    ddy_filtered = applyDeadzone(ddy_temp, noise_margin);
    ddz_filtered = applyDeadzone(ddz_temp, noise_margin);
end

function val_filtered = applyDeadzone(val, margin)
    % Ensure that the function outputs the same type as the input
    if abs(val) < margin
        val_filtered = cast(0, 'like', val); % Cast zero to the type of val
    else
        val_filtered = val;
    end
end

== matlab function flightControlSystem/Control System/Controller/Position Controller/Position error transformation (Earth to Body frame)3 ==
  data: yaw input; xy_err_earth input; xy_err_body output
function xy_err_body = fcn(yaw,xy_err_earth)

transformation = [cos(yaw), sin(yaw); -sin(yaw),  cos(yaw)];
xy_err_body = transformation * xy_err_earth;


end

== matlab function flightControlSystem/Image Processing System/MATLAB Function4 ==
  data: u input; forward output; right output; yawgo output; left output; sum_of_region_right output; sum_of_region_forward output; yawcheck output
function [forward,right,yawgo,left,sum_of_region_right,sum_of_region_forward,yawcheck]= fcn(u)



    
        
        % Determine the midpoint of the image along the vertical axis
   
        
        % Set the pixels below the midpoint to black
        %u(midpoint + 10:end, :) = 0;
        
        % Perform noise reduction
        
%         if (filtered_u(1:30,75:85))==1
%             forward=1
%             right=0
%         elseif (filtered_u(58:65,120:150))==1
%             forward=0
%             right=1
%         else
%             forward=0
%             right=0
%         end

%%%%%%%%%%%%%%%%%%%%%%%%%%%%%%%%%%%%%%%%%%%%%%%%%%%%%%%%
        row_range_right = 55:65;
        col_range_right = 90:150;
   
        region_of_interest_right = u(row_range_right, col_range_right);
  
        sum_of_region_right = sum(region_of_interest_right(:))

        %%%%%%%%%%%%%%%%%%%%%%%%%%%%%%%%%%%%%%%%%%%%%%%%%%%%%%
         row_range_forward = 1:70;
         col_range_forward = 75:85;
        
         region_of_interest_forward = u(row_range_forward, col_range_forward);
        
         sum_of_region_forward = sum(region_of_interest_forward(:))


         %%%%%%%%%%%%%%%%%%%%%%%%%%%%%%%%%%%%%%%%%%%%%%%%%%%%%

         row_range_left=55:65;
         col_range_left=1:90;
         region_of_interest_left = u(row_range_left, col_range_left);
        
         sum_of_region_left = sum(region_of_interest_left(:))


%%%%%%%%%%%%%%%%%%%%%%%%%%%%%%%%%%%%%%%%%%%%%%%%%%%%%%
        mid_area=u(59:61,78:82);
        yawcheck=sum(mid_area(:))
        if yawcheck>12
            yawgo=1
        else
            yawgo=0
        end




        %%%%%%%%%%%%%%%%%%%%%%%%%%%%%%%%%%%%%%%%%
%         if u(48:50,80:82)==1 
%             circle_area1=1;
%         else
%             circle_area1=0;
%         end
%       
%         if u(80:82:80:82)==1
%             circle_area2=1
%         else
%             circle_area2=0
%         end
% 
%         if circle_area2 && circle_area1==1
% 
%             land=1;
%         else
%             land=0;
%         end

%%%%%%%%%%%%%%%%%%%%%%%%%%%%%%%%%%%%%%%%%%%%%%%%

        if sum_of_region_right>160
               right=1;
               forward=0;
               left=0;
  
        elseif sum_of_region_forward>190
            forward=1;
            right=0;
            left=0;

        elseif sum_of_region_left>170
            left=1;
            forward=0;
            right=0;
        else
            forward=0;
            right=0;
            left=0;
        end


%         % Define the region of interest for circle detection
%         row_range_circle = [40:80]; 
%         col_range_circle = [60:100]; 
%     
%         % Extract the region of interest for circle detection
%         region_of_interest_circle = u(row_range_circle, col_range_circle);
%     
%         % Calculate the center and radius of the circle
%         center = [length(row_range_circle)/2, length(col_range_circle)/2];
%         radius = min(length(row_range_circle), length(col_range_circle)) / 2;
%     
%         % Generate a circle using the equation of a circle
%         [x, y] = meshgrid(1:length(col_range_circle), 1:length(row_range_circle));
%         circle = (x - center(2)).^2 + (y - center(1)).^2 <= radius^2;
%     
%         % Compare the region of interest with the generated circle
%         similarity = sum(sum(region_of_interest_circle & circle)) / sum(circle(:))
% 
%     
%         % Set a threshold for circle detection (adjust as needed)
%         threshold = 0.7;
%     
%         % If the region of interest is similar to the generated circle, set the land flag
%         if similarity > threshold
%             land = 1
%         else
%             land=0
%         end
end

== matlab function flightControlSystem/Control System/Controller/Position Controller/MATLAB Function ==
  data: pid_input input; filtered_output output; filtered_output2 output
function [filtered_output, filtered_output2] = removeSmallAmplitude(pid_input)
    % This function removes elements from the PID input where the absolute
    % amplitude is less than 0.01.

    % Define the threshold
    threshold = 0.001;
    
    % Initialize outputs
    filtered_output = single(0);  % Change 'single' to 'double' if required
    filtered_output2 = single(0);  % Change 'single' to 'double' if required
    
    % Check and assign values based on condition
    if abs(pid_input(1)) > threshold
        filtered_output = single(pid_input(1));  % Ensure type consistency
      
        filtered_output2 = single(pid_input(2));  % Ensure type consistency
       
    end
end

== stateflow chart flightControlSystem/Control System/Path Planning/yaw ==
  state hover10 [commented out]
    xout = xout;
    yout = yout-0.0002;
    zout = -0.7;
  state land5 [commented out]
    xout =xout;
    yout = yout ;
    zout = -0.7;
    finaland=1
  state hover9 [commented out]
    xout = xout-0.0001;
    yout = yout;
    zout = -0.7;
    yaw=yaw
  state right1 [commented out]
    xout =xout;
    yout = yout-0.0005 ;
    zout = -0.7;
  state land4 [commented out]
    xout =xout;
    yout = yout ;
    zout = -0.7;
  state land3 [commented out]
    xout =xout;
    yout = yout ;
    zout = -0.7;
  state land
    xout =xout;
    yout = yout ;
    zout = -0.5;
  state hover11 [commented out]
    xout = xout;
    yout = yout;
    zout = -0.7;
  state hover12
    xout =xout;
    yout = yout ;
    zout = -0.5;
  state hover4
    xout = xout-0.0001;
    yout = yout;
    zout = -0.5;
    yaw=yaw
  state hover7
    xout = xout;
    yout = yout+0.0003;
    zout = -0.5;
  state hover14
    xout = xout;
    yout = yout+0.0005;
    zout = -0.5;
  state right
    xout =xout;
    yout = yout ;
    zout = -0.5;
    yaw=yaw+0.0007
  state hover8
    xout = xout;
    yout = yout;
    zout = -0.5;
  state land6
    xout =xout;
    yout = yout ;
    zout = -0.7;
  state hover13
    xout =xout;
    yout = yout ;
    zout = -0.5;
  state go
    xout = xout + 0.0005;
    yout = yout ;
    zout = -0.5;
  state land1
    xout =xout;
    yout = yout ;
    zout = -0.7;
    finaland=1
  state hover3
    xout = xout;
    yout = yout;
    zout = -0.5;
  state hover
    xout = 0.0;
    yout = 0.0;
    zout = -0.7;
    yaw=0.0
  state search
    xout = xout;
    yout = yout+0.0002 ;
    zout = -0.7;
  state hover5
    xout = xout;
    yout = yout;
    zout = -0.7;
  state hover1
    xout = xout;
    yout = yout;
    zout = -0.7;
  state searchforward
    xout = xout + 0.0004;
    yout = yout ;
    zout = -0.7;
  state search1
    xout = xout ;
    yout = yout -0.0002;
    zout = -0.7;
  state yawalign1
    xout = xout ;
    yout = yout ;
    zout = -0.5;
    yaw=yaw+0.0003
  state hover6
    xout = xout;
    yout = yout;
    zout = -0.7;
  state yawalign
    xout = xout ;
    yout = yout ;
    zout = -0.5;
    yaw=yaw-0.0003
  state hover2
    xout = xout;
    yout = yout;
    zout = -0.7;
  land3 -> hover10 [commented out] : [after(2,sec)&&land==0]
  hover10 -> land5 [commented out] : [land==1]
  land3 -> land5 [commented out] : [after(2,sec)&&land==1]
  land4 -> right1 [commented out]
  right1 -> land3 [commented out] : [land==1]
  hover9 -> land4 [commented out] : [left==1]
  hover11 -> hover9 [commented out] : after(2,sec)
  land -> hover7 : [forward==0&&yawgo==1]
  go -> hover11 [commented out] : [after(5,sec)&&left==1]
  hover14 -> land : [after(8,sec)&&forward==0&&yawgo==0]
  hover4 -> hover12 : [right==1&& yawgo==1]
  hover12 -> right : [right==1&&yawgo==1]
  hover8 -> hover4 : after(2,sec)
  hover7 -> land6 : [after(2,sec)&&yawgo==1&&forward==0]
  hover13 -> hover14 : after(2,sec)
  right -> hover13 : [yawgo==1&&forward==1]
  hover -> hover8 [order 1] : [after(5,sec)&&right==1]
  land6 -> land1 : [after(2,sec)&&yawgo==1&&forward==0]
  go -> hover8 : [ right==1&&forward==0]
  hover3 -> go : after(3,sec)
  hover -> go [order 3] : [after(5, sec) && forward==1]
  search1 -> hover3 [order 1] : [after(5,sec)&&forward==1]
  yawalign -> hover3 [order 1] : [after(3.5,sec)&&forward==1]
  (default) -> hover
  yawalign1 -> hover3 [order 1] : [after(3.5,sec)&&forward==1]
  searchforward -> hover3 [order 1] : [after(5,sec)&&forward==1]
  search -> hover3 [order 1] : [after(5,sec)&&forward==1]
  hover -> searchforward [order 2] : [after(8, sec) && forward==0 && right==0]
  search -> hover1 [order 2] : [after(7,sec) &&forward==0&&yawgo==0]
  hover5 -> search : after(3,sec)
  searchforward -> hover5 [order 2] : [after(5,sec)&&forward==0&&yawgo==0]
  hover1 -> search1 [order 1] : [after(2,sec)&&forward==0&&yawgo==0]
  search -> hover6 [order 3] : [yawgo==1&&forward==0]
  hover2 -> search [order 1] : [after(3,sec)&&forward==0&&yawgo==0]
  hover1 -> hover2 [order 2] : [yawgo==1]
  yawalign -> searchforward [order 2] : [after(5,sec)&&yawgo==0&&forward==0]
  searchforward -> hover6 [order 3] : [yawgo==1&&forward==0]
  yawalign -> yawalign1 [order 3] : [yaw<-0.9&&forward==0&&yawgo==1]
  yawalign1 -> yawalign [order 2] : [yaw>0.9&&forward==0&&yawgo==1]
  search1 -> hover6 [order 3] : [yawgo==1&&forward==0]
  search1 -> hover2 [order 2] : [after(12,sec)&&forward==0&&yawgo==0]
  hover6 -> yawalign : after(2,sec)
  hover2 -> hover6 [order 2] : [after(2,sec)&&yawgo==1]
  data: yawgo input; xout output; yout output; forward input; right input; yaw output; finaland output; left input; zout output double

== matlab function flightControlSystem/Control System/Controller/Position Controller/Subsystem/Position error transformation (Earth to Body frame) ==
  data: yaw input; xy_err_earth input; xy_err_body output
function xy_err_body = fcn(yaw,xy_err_earth)

transformation = [cos(yaw), sin(yaw); -sin(yaw),  cos(yaw)];
xy_err_body = transformation * xy_err_earth;


end

== stateflow chart flightControlSystem/Control System/Path Planning/Path Planning/Chart ==
  settings: initializeOutput=1
  state hover4
    xout = xout-0.0005;
    yout = yout;
    zout = -0.7;
  state right
    xout =xout;
    yout = yout+0.001 ;
    zout = -0.7;
  state go
    xout = xout + 0.003;
    yout = yout ;
    zout = -0.7;
  state hover
    xout = 0.0;
    yout = 0.0;
    zout = -1.0;
  state hover3
    xout = xout;
    yout = yout;
    zout = -0.7;
  state search1
    xout = xout ;
    yout = yout +0.005;
    zout = -0.7;
  state search
    xout = xout;
    yout = yout-0.005 ;
    zout = -0.7;
  state hover6
    xout = xout;
    yout = yout;
    zout = -0.7;
  state hover2
    xout = xout;
    yout = yout;
    zout = -0.7;
  hover4 -> right : [after(1,sec)&&right==1]
  go -> hover4 : [ right==1&&forward==0]
  (default) -> hover
  hover -> go [order 2] : [after(5, sec) && forward==1]
  hover3 -> go : after(3,sec)
  search1 -> hover3 [order 1] : [forward==1]
  hover -> search [order 1] : [after(5, sec) && forward==0]
  search -> hover3 [order 1] : [forward==1]
  hover6 -> search1 : [after(2,sec)&&forward==0]
  search -> hover6 [order 2] : [after(3,sec) &&forward==0]
  search1 -> hover2 [order 2] : [after(3,sec)&&forward==0]
  hover2 -> search : [after(3,sec)&&forward==0]
  data: xout output; yout output; zout output; forward input; right input

== matlab function flightControlSystem/Control System/Path Planning/MATLAB Function ==
  data: u input; forward output; right output
function [forward,right]= fcn(u)

forward = u(1);
right=u(2);
